simulink model "Experiment_3_cs"  (Simulink 8.4)
settings: Solver=ode5  SolverMode=SingleTasking  StartTime=0.0  StopTime=inf  FixedStep=1/100  RelTol=1e-3
PreLoadFcn:
  | mbxruntime.callbacks.PreLoadFcn(bdroot);
PostLoadFcn:
  | mbxruntime.callbacks.PostLoadFcn(bdroot);
InitFcn:
  | mbxruntime.callbacks.InitFcn(bdroot);
StartFcn:
  | mbxruntime.callbacks.StartFcn(bdroot);
StopFcn:
  | mbxruntime.callbacks.StopFcn(bdroot);
undefined symbols (not defined in the file or in its folder): dfreq, gray, Rec, SDTV, strel
libraries: simulink x88, PreScanSimulinkLibrary x24, simulink_extras x22, visiontextngfix x15, visionconversions x3, PreScanUsefulBlocks x3, visionsinks x2, simulink_need_slupdate x2, visionstatistics x1, visionmorphops x1, visionanalysis x1
(part 5 of 12)

== system Experiment_3_cs/SELF_Audi_A8_1/DISABLED/GND1 ==
  GND_Alt : Constant  Value=0
  GND_Lat : Constant  Value=0
  GND_Long : Constant  Value=0
  GND_OrientationPitch : Constant  Value=0
  GND_OrientationRoll : Constant  Value=0
  GND_OrientationYaw : Constant  Value=0
  GND_PositionX : Constant  Value=0
  GND_PositionY : Constant  Value=0
  GND_PositionZ : Constant  Value=0
  GND_Velocity : Constant  Value=0
  GND_Yaw_rate : Constant  Value=0
  buscreator : BusCreator  Inputs=11  OutDataTypeStr=Bus: PRESCAN_SELFSENSORDATA  NonVirtualBus=on
  bus : Outport  OutDataTypeStr=Bus: PRESCAN_SELFSENSORDATA
  wires:
  GND_PositionX/1 -> buscreator/1  "PositionX"
  GND_PositionY/1 -> buscreator/2  "PositionY"
  GND_PositionZ/1 -> buscreator/3  "PositionZ"
  GND_OrientationRoll/1 -> buscreator/4  "OrientationRoll"
  GND_OrientationPitch/1 -> buscreator/5  "OrientationPitch"
  GND_OrientationYaw/1 -> buscreator/6  "OrientationYaw"
  GND_Velocity/1 -> buscreator/7  "Velocity"
  GND_Yaw_rate/1 -> buscreator/8  "Yaw_rate"
  GND_Lat/1 -> buscreator/9  "Lat"
  GND_Long/1 -> buscreator/10  "Long"
  GND_Alt/1 -> buscreator/11  "Alt"
  buscreator/1 -> bus/1

== system Experiment_3_cs/SELF_BMW_Z3_1/DISABLED/GND1 ==
  GND_Alt : Constant  Value=0
  GND_Lat : Constant  Value=0
  GND_Long : Constant  Value=0
  GND_OrientationPitch : Constant  Value=0
  GND_OrientationRoll : Constant  Value=0
  GND_OrientationYaw : Constant  Value=0
  GND_PositionX : Constant  Value=0
  GND_PositionY : Constant  Value=0
  GND_PositionZ : Constant  Value=0
  GND_Velocity : Constant  Value=0
  GND_Yaw_rate : Constant  Value=0
  buscreator : BusCreator  Inputs=11  OutDataTypeStr=Bus: PRESCAN_SELFSENSORDATA  NonVirtualBus=on
  bus : Outport  OutDataTypeStr=Bus: PRESCAN_SELFSENSORDATA
  wires:
  GND_PositionX/1 -> buscreator/1  "PositionX"
  GND_PositionY/1 -> buscreator/2  "PositionY"
  GND_PositionZ/1 -> buscreator/3  "PositionZ"
  GND_OrientationRoll/1 -> buscreator/4  "OrientationRoll"
  GND_OrientationPitch/1 -> buscreator/5  "OrientationPitch"
  GND_OrientationYaw/1 -> buscreator/6  "OrientationYaw"
  GND_Velocity/1 -> buscreator/7  "Velocity"
  GND_Yaw_rate/1 -> buscreator/8  "Yaw_rate"
  GND_Lat/1 -> buscreator/9  "Lat"
  GND_Long/1 -> buscreator/10  "Long"
  GND_Alt/1 -> buscreator/11  "Alt"
  buscreator/1 -> bus/1

== system Experiment_3_cs/SELF_Male_RegularAni_1/DISABLED/GND1 ==
  GND_Alt : Constant  Value=0
  GND_Lat : Constant  Value=0
  GND_Long : Constant  Value=0
  GND_OrientationPitch : Constant  Value=0
  GND_OrientationRoll : Constant  Value=0
  GND_OrientationYaw : Constant  Value=0
  GND_PositionX : Constant  Value=0
  GND_PositionY : Constant  Value=0
  GND_PositionZ : Constant  Value=0
  GND_Velocity : Constant  Value=0
  GND_Yaw_rate : Constant  Value=0
  buscreator : BusCreator  Inputs=11  OutDataTypeStr=Bus: PRESCAN_SELFSENSORDATA  NonVirtualBus=on
  bus : Outport  OutDataTypeStr=Bus: PRESCAN_SELFSENSORDATA
  wires:
  GND_PositionX/1 -> buscreator/1  "PositionX"
  GND_PositionY/1 -> buscreator/2  "PositionY"
  GND_PositionZ/1 -> buscreator/3  "PositionZ"
  GND_OrientationRoll/1 -> buscreator/4  "OrientationRoll"
  GND_OrientationPitch/1 -> buscreator/5  "OrientationPitch"
  GND_OrientationYaw/1 -> buscreator/6  "OrientationYaw"
  GND_Velocity/1 -> buscreator/7  "Velocity"
  GND_Yaw_rate/1 -> buscreator/8  "Yaw_rate"
  GND_Lat/1 -> buscreator/9  "Lat"
  GND_Long/1 -> buscreator/10  "Long"
  GND_Alt/1 -> buscreator/11  "Alt"
  buscreator/1 -> bus/1

== system Experiment_3_cs/SELF_Nissan_Cabstar_1/DISABLED/GND1 ==
  GND_Alt : Constant  Value=0
  GND_Lat : Constant  Value=0
  GND_Long : Constant  Value=0
  GND_OrientationPitch : Constant  Value=0
  GND_OrientationRoll : Constant  Value=0
  GND_OrientationYaw : Constant  Value=0
  GND_PositionX : Constant  Value=0
  GND_PositionY : Constant  Value=0
  GND_PositionZ : Constant  Value=0
  GND_Velocity : Constant  Value=0
  GND_Yaw_rate : Constant  Value=0
  buscreator : BusCreator  Inputs=11  OutDataTypeStr=Bus: PRESCAN_SELFSENSORDATA  NonVirtualBus=on
  bus : Outport  OutDataTypeStr=Bus: PRESCAN_SELFSENSORDATA
  wires:
  GND_PositionX/1 -> buscreator/1  "PositionX"
  GND_PositionY/1 -> buscreator/2  "PositionY"
  GND_PositionZ/1 -> buscreator/3  "PositionZ"
  GND_OrientationRoll/1 -> buscreator/4  "OrientationRoll"
  GND_OrientationPitch/1 -> buscreator/5  "OrientationPitch"
  GND_OrientationYaw/1 -> buscreator/6  "OrientationYaw"
  GND_Velocity/1 -> buscreator/7  "Velocity"
  GND_Yaw_rate/1 -> buscreator/8  "Yaw_rate"
  GND_Lat/1 -> buscreator/9  "Lat"
  GND_Long/1 -> buscreator/10  "Long"
  GND_Alt/1 -> buscreator/11  "Alt"
  buscreator/1 -> bus/1

== system Experiment_3_cs/TIS_1/DISABLED/GND1 ==
  GND_DATA : Subsystem
  GND_HEADER : Subsystem
  buscreator : BusCreator  Inputs=2  OutDataTypeStr=Bus: PRESCAN_SCANNERSENSOR_MESSAGE  NonVirtualBus=on
  concatenate : Concatenate  NumInputs=5
  bus : Outport  OutDataTypeStr=Bus: PRESCAN_SCANNERSENSOR_MESSAGE
  wires:
  GND_HEADER/1(bus) -> buscreator/1  "HEADER"
  GND_DATA/1(bus) -> buscreator/2  "DATA"
  buscreator/1 -> concatenate/1, concatenate/2, concatenate/3, concatenate/4, concatenate/5
  concatenate/1 -> bus/1

== system Experiment_3_cs/TIS_2/DISABLED/GND1 ==
  GND_DATA : Subsystem
  GND_HEADER : Subsystem
  buscreator : BusCreator  Inputs=2  OutDataTypeStr=Bus: PRESCAN_SCANNERSENSOR_MESSAGE  NonVirtualBus=on
  concatenate : Concatenate  NumInputs=5
  bus : Outport  OutDataTypeStr=Bus: PRESCAN_SCANNERSENSOR_MESSAGE
  wires:
  GND_HEADER/1(bus) -> buscreator/1  "HEADER"
  GND_DATA/1(bus) -> buscreator/2  "DATA"
  buscreator/1 -> concatenate/1, concatenate/2, concatenate/3, concatenate/4, concatenate/5
  concatenate/1 -> bus/1

== system Experiment_3_cs/Actros_2541_1/ENABLED/Dynamics_Empty/MuxState ==
  note: mode: Dynamics
  note: mode: Positioning
  note: mode: Dynamics
      | VelVEHICLE
      | wrt VEH
  note: AnglesVEHICLE
      | wrtGLOB
  note: For state mode 'Dynamic' positions
      | are not taken into account, as they
      | are computed by integrating velocity.
      | Click annotation for Help.
  x [m] : Inport  SampleTime=TimeStep
  y [m] : Inport  Port=2  SampleTime=TimeStep
  z [m] : Inport  Port=3  SampleTime=TimeStep
  dx [m/s] : Inport  Port=4  SampleTime=TimeStep
  dy [m/s] : Inport  Port=5  SampleTime=TimeStep
  dz [m/s] : Inport  Port=6  SampleTime=TimeStep
  R [rad] : Inport  Port=7  SampleTime=TimeStep
  P [rad] : Inport  Port=8  SampleTime=TimeStep
  Y [rad] : Inport  Port=9  SampleTime=TimeStep
  Constant : Constant  DisableCoverage=on  Value=positioningmode
  Discrete-Time Integrator : DiscreteIntegrator  SampleTime=TimeStep
  Ground : Ground
  Ground1 : Ground
  Mux1 : Mux  Inputs=[3 3]
  Mux2 : Mux  Inputs=3
  Mux3 : Mux  Inputs=3
  Mux4 : Mux  Inputs=3
  Mux5 : Mux  Inputs=[3 3]
  Mux6 : Mux  Inputs=[6 3]
  Switch : Switch  Threshold=0.5
  Transformation_BODY2GLOBAL : PreScanSimulinkLibrary/Simple_Vehicle_Dynamics/Chassis/MuxDynState/Transformation_BODY2GLOBAL
  mux3 : Mux  Inputs=3
  state : Outport
  wires:
  Constant/1 -> Switch/2
  Mux6/1 -> state/1
  Mux4/1 -> Mux1/1
  Mux5/1 -> Switch/3
  Mux1/1 -> Switch/1
  Switch/1 -> Mux6/1  "PosVeh wrt  GLOB"
  P [rad]/1 -> Mux3/2
  R [rad]/1 -> Mux3/1
  dz [m/s]/1 -> Mux2/3
  dy [m/s]/1 -> Mux2/2
  dx [m/s]/1 -> Mux2/1
  z [m]/1 -> Mux4/3
  y [m]/1 -> Mux4/2
  x [m]/1 -> Mux4/1
  Ground1/1 -> mux3/2  "pitch"
  Y [rad]/1 -> mux3/3, Mux3/3  "yaw"
  Mux3/1 -> Mux6/2
  Transformation_BODY2GLOBAL/1 -> Discrete-Time Integrator/1, Mux5/2  "VelVEH wrt  GLOB"
  mux3/1 -> Transformation_BODY2GLOBAL/2
  Ground/1 -> mux3/1  "roll"
  Mux2/1 -> Mux1/2, Transformation_BODY2GLOBAL/1
  Discrete-Time Integrator/1 -> Mux5/1  "PosVEH wrt  GLOB"

== system Experiment_3_cs/Actros_2541_1/ENABLED/SELF_Demux/compas converter ==
  rotz [rad] : Inport
  cart2compas : Subsystem
  rad2deg : Gain  Gain=180/pi
  heading [deg] : Outport
  wires:
  rad2deg/1 -> cart2compas/1(Angle [deg])
  rotz [rad]/1 -> rad2deg/1
  cart2compas/1(heading [deg]) -> heading [deg]/1

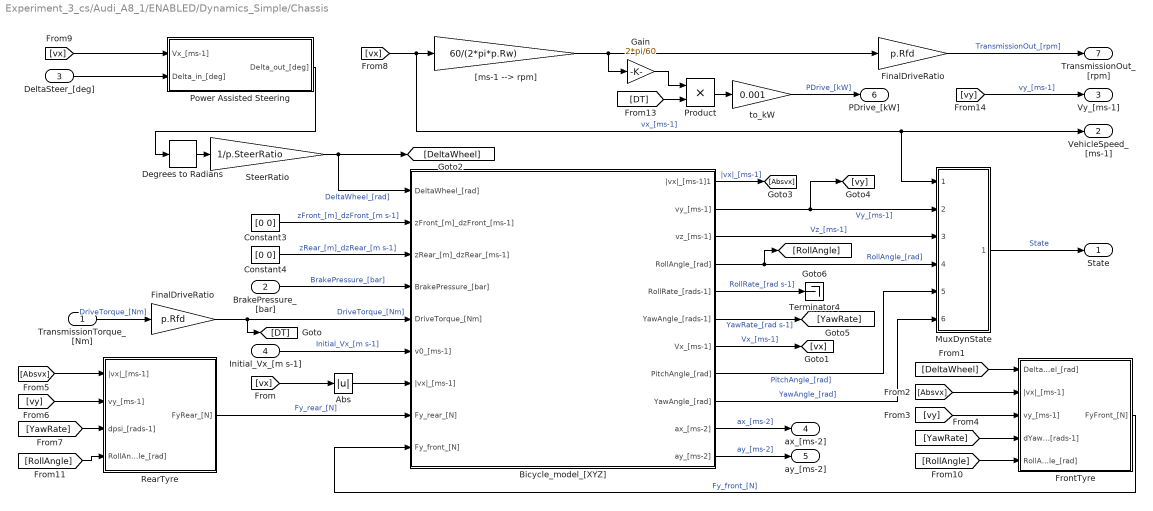
== system Experiment_3_cs/Audi_A8_1/ENABLED/Dynamics_Simple/Chassis ==
  TransmissionTorque_[Nm] : Inport
  BrakePressure_[bar] : Inport  Port=2
  DeltaSteer_[deg] : Inport  Port=3
  Initial_Vx_[m s-1] : Inport  Port=4
  Abs : Abs
  Bicycle_model_[XYZ] : Subsystem
      mask Display: image(imread('Bicycle_model.png'));
  Constant3 : Constant  Value=[0 0]
  Constant4 : Constant  Value=[0 0]
  Degrees to Radians : simulink_extras/Transformations/Degrees to Radians
  FinalDriveRatio : Gain  Gain=p.Rfd  SaturateOnIntegerOverflow=on  OutDataTypeStr=Inherit: Same as input  ParamDataTypeStr=Inherit: Same as input
  "FinalDriveRatio " : Gain  Gain=p.Rfd  SaturateOnIntegerOverflow=on  OutDataTypeStr=Inherit: Same as input  ParamDataTypeStr=Inherit: Same as input
  FrontTyre : Subsystem
      mask Display: image(imread('Tyre.png'));
  Gain : Gain  Gain=2*pi/60
  MuxDynState : Subsystem
  Power Assisted Steering : Subsystem
  Product : Product  RndMeth=Zero
  RearTyre : Subsystem
      mask Display: image(imread('Tyre.png'));
  SteerRatio : Gain  Gain=1/p.SteerRatio
  Terminator4 : Terminator
  "[ms-1 --> rpm]" : Gain  Gain=60/(2*pi*p.Rw)  SaturateOnIntegerOverflow=on  OutDataTypeStr=Inherit: Same as input  ParamDataTypeStr=Inherit: Same as input
  to_kW : Gain  Gain=0.001
  State : Outport
  VehicleSpeed_[ms-1] : Outport  Port=2
  Vy_[ms-1] : Outport  Port=3
  ax_[ms-2] : Outport  Port=4
  ay_[ms-2] : Outport  Port=5
  PDrive_[kW] : Outport  Port=6
  TransmissionOut_[rpm] : Outport  Port=7
  wires:
  [vy] -> Vy_[ms-1]/1  "vy_[ms-1]"
  to_kW/1 -> PDrive_[kW]/1  "PDrive_[kW]"
  Gain/1 -> Product/1
  Bicycle_model_[XYZ]/10(ax_[ms-2]) -> ax_[ms-2]/1  "ax_[ms-2]"
  Product/1 -> to_kW/1
  [DT] -> Product/2
  Bicycle_model_[XYZ]/11(ay_[ms-2]) -> ay_[ms-2]/1  "ay_[ms-2]"
  Abs/1 -> Bicycle_model_[XYZ]/7(|vx|_[ms-1])
  Degrees to Radians/1 -> SteerRatio/1
  [vx] -> Abs/1
  SteerRatio/1 -> [DeltaWheel], Bicycle_model_[XYZ]/1(DeltaWheel_[rad])  "DeltaWheel_[rad]"
  TransmissionTorque_[Nm]/1 -> "FinalDriveRatio "/1  "DriveTorque_[Nm]"
  RearTyre/1(FyRear_[N]) -> Bicycle_model_[XYZ]/8(Fy_rear_[N])  "Fy_rear_[N]"
  FrontTyre/1(FyFront_[N]) -> Bicycle_model_[XYZ]/9(Fy_front_[N])  "Fy_front_[N]"
  Bicycle_model_[XYZ]/1(|vx|_[ms-1]1) -> [Absvx]  "|vx|_[ms-1]"
  Bicycle_model_[XYZ]/2(vy_[ms-1]) -> [vy], MuxDynState/2(vy [ms-1])  "Vy_[ms-1]"
  Bicycle_model_[XYZ]/4(RollAngle_[rad]) -> MuxDynState/4(R [rad]), [RollAngle]  "RollAngle_[rad]"
  Bicycle_model_[XYZ]/6(YawAngle_[rads-1]) -> [YawRate]  "YawRate_[rad s-1]"
  Bicycle_model_[XYZ]/7(Vx_[ms-1]) -> [vx]  "Vx_[ms-1]"
  [DeltaWheel] -> FrontTyre/1(DeltaWheel_[rad])
  [Absvx] -> FrontTyre/2(|vx|_[ms-1])
  [vy] -> FrontTyre/3(vy_[ms-1])
  [YawRate] -> FrontTyre/4(dYawAngle_[rads-1])
  [Absvx] -> RearTyre/1(|vx|_[ms-1])
  [vy] -> RearTyre/2(vy_[ms-1])
  [YawRate] -> RearTyre/3(dpsi_[rads-1])
  Bicycle_model_[XYZ]/3(vz_[ms-1]) -> MuxDynState/3(vz [ms-1])  "Vz_[ms-1]"
  Bicycle_model_[XYZ]/8(PitchAngle_[rad]) -> MuxDynState/5(P [rad])  "PitchAngle_[rad]"
  Bicycle_model_[XYZ]/9(YawAngle_[rad]) -> MuxDynState/6(Y [rad])  "YawAngle_[rad]"
  "[ms-1 --> rpm]"/1 -> Gain/1, FinalDriveRatio/1
  FinalDriveRatio/1 -> TransmissionOut_[rpm]/1  "TransmissionOut_[rpm]"
  [vx] -> "[ms-1 --> rpm]"/1, VehicleSpeed_[ms-1]/1, MuxDynState/1(vx [ms-1])  "vx_[ms-1]"
  [vx] -> Power Assisted Steering/1(Vx_[ms-1])
  DeltaSteer_[deg]/1 -> Power Assisted Steering/2(Delta_in_[deg])
  Power Assisted Steering/1(Delta_out_[deg]) -> Degrees to Radians/1
  [RollAngle] -> FrontTyre/5(RollAngle_[rad])
  [RollAngle] -> RearTyre/4(RollAngle_[rad])
  Constant3/1 -> Bicycle_model_[XYZ]/2(zFront_[m]_dzFront_[ms-1])  "zFront_[m]_dzFront_[m s-1]"
  Constant4/1 -> Bicycle_model_[XYZ]/3(zRear_[m]_dzRear_[ms-1])  "zRear_[m]_dzRear_[m s-1]"
  BrakePressure_[bar]/1 -> Bicycle_model_[XYZ]/4(BrakePressure_[bar])  "BrakePressure_[bar]"
  "FinalDriveRatio "/1 -> Bicycle_model_[XYZ]/5(DriveTorque_[Nm]), [DT]  "DriveTorque_[Nm]"
  Initial_Vx_[m s-1]/1 -> Bicycle_model_[XYZ]/6(v0_[ms-1])  "Initial_Vx_[m s-1]"
  Bicycle_model_[XYZ]/5(RollRate_[rads-1]) -> Terminator4/1  "RollRate_[rad s-1]"
  MuxDynState/1(State) -> State/1  "State"

== system Experiment_3_cs/Audi_A8_1/ENABLED/Dynamics_Simple/Engine ==
  ImpellerTorque_[Nm] : Inport
  Throttle_[%] : Inport  Port=2
  Configurable Subsystem : Subsystem  BlockChoice=Rate Limiter  mask{ComputationMode=ComputationMode}
      mask prompts: ComputationMode "Compuation mode:"
      mask init:
      | SetComputationMode(gcb,ComputationMode);
      settings: AttributesFormatString=%<BlockChoice>  OpenFcn=BringToFront(gcb);  MemberBlocks=Discrete Rate Limiter,Rate Limiter
      settings: TemplateBlock=|
      | PreScanSimulinkLibrary/Configurable Subsystems/TransferFunction
      | Engine/Configurable
      | Subsystem
  Configurable Subsystem1 : Subsystem  BlockChoice=Integrator  mask{ComputationMode=ComputationMode}
      mask prompts: ComputationMode "Computation mode:"
      mask init:
      | SetComputationMode(gcb,ComputationMode);
      settings: AttributesFormatString=%<BlockChoice>  OpenFcn=BringToFront(gcb);  MemberBlocks=Discrete-Time Integrator,Integrator
      settings: TemplateBlock=|
      | PreScanSimulinkLibrary/Configurable Subsystems/integral with initial condition and limts
      | for engine/Configurable
      | Subsystem
  EngineTorque : Lookup2D  RowIndex=p.thvec  ColumnIndex=p.nevec  Table=p.emap  InputSameDT=on
  Gain : Gain  Gain=2*pi/60
  Product : Product  RndMeth=Zero
  Sum : Sum  Inputs=-+  SaturateOnIntegerOverflow=on  InputSameDT=on  OutDataTypeStr=Inherit: Same as first input
  engine + impeller inertia : Gain  Gain=1/p.Iei  SaturateOnIntegerOverflow=on  OutDataTypeStr=Inherit: Same as input  ParamDataTypeStr=Inherit: Same as input
  to_kW : Gain  Gain=0.001
  nEngine_[rpm] : Outport  InitialOutput=0
  PEngine_[kW] : Outport  Port=2  InitialOutput=0
  wires:
  EngineTorque/1 -> Sum/2, Product/2
  engine + impeller inertia/1 -> Configurable Subsystem1/1(In1)
  Sum/1 -> engine + impeller inertia/1
  Configurable Subsystem1/1(Out1) -> nEngine_[rpm]/1, EngineTorque/2, Gain/1  "rpm"
  Throttle_[%]/1 -> Configurable Subsystem/1(In1)
  ImpellerTorque_[Nm]/1 -> Sum/1
  Configurable Subsystem/1(Out1) -> EngineTorque/1
  Product/1 -> to_kW/1
  Gain/1 -> Product/1
  to_kW/1 -> PEngine_[kW]/1

== system Experiment_3_cs/Audi_A8_1/ENABLED/Dynamics_Simple/Gear: Auto Manual ==
  note: 0; Auto = on // Manual =off
      | 1; Auto = off // Manual =on
  Auto_Manual : Inport
  Manual_Gear : Inport  Port=2
  Auto_Gear : Inport  Port=3
  If : If  IfExpression=u1 == 0
  If Action Subsystem : Subsystem  TreatAsAtomicUnit=on
  If Action Subsystem1 : Subsystem  TreatAsAtomicUnit=on
  Merge : Merge
  Gear : Outport
  wires:
  If Action Subsystem/1(Out1) -> Merge/1
  Auto_Gear/1 -> If Action Subsystem/1(In1)
  If/1 -> If Action Subsystem/Action
  Merge/1 -> Gear/1
  If Action Subsystem1/1(Out1) -> Merge/2
  Manual_Gear/1 -> If Action Subsystem1/1(In1)
  If/2 -> If Action Subsystem1/Action
  Auto_Manual/1 -> If/1

== system Experiment_3_cs/Audi_A8_1/ENABLED/Dynamics_Simple/ShiftLogic ==
  Throttle_[%] : Inport
  GearNr_[-] : Inport  Port=2
  Auto_GearShift : Inport  Port=3
  VehSpeed_[ms-1] : Inport  Port=4
  Add2 : Sum
  Data Type Conversion1 : DataTypeConversion  OutDataTypeStr=double
  Detect Increase1 : simulink/Logic and Bit Operations/Detect Increase  vinit=0.0  InputProcessing=Inherited  OutDataTypeStr=uint8
  Detect Increase : Subsystem
  Gear limitation : Saturate  UpperLimit=p.maxGear  LowerLimit=1
  Gear limitation while shifting : Saturate  UpperLimit=p.maxGear  LowerLimit=1
  GearNeutral : Constant  Value=0
  GearReverse : Constant  Value=-1
  "IC, gear = 1" : Memory  X0=1  InheritSampleTime=on
  If Action Neutral : Subsystem  TreatAsAtomicUnit=on
  If Action Normal : Subsystem  TreatAsAtomicUnit=on
  If Action Reverse : Subsystem  TreatAsAtomicUnit=on
  Memory : Memory  InheritSampleTime=on
  Merge : Merge  Inputs=3
  Relational Operator : RelationalOperator  OutDataTypeStr=boolean
  Relational Operator1 : RelationalOperator  Operator=<=  OutDataTypeStr=boolean
  Shift_Down time : Delay  DelayLength=p.ShiftDown_fac  InputProcessing=Inherited
  Shift_Up time : Delay  DelayLength=p.ShiftUp_fac  InputProcessing=Inherited
  Sum : Sum  Inputs=+-
  interp_down : Lookup2D  RowIndex=p.downth  ColumnIndex=[1:p.maxGear]  Table=p.downtab  LookUpMeth=Interpolation-Use End Values  InputSameDT=on
  interp_up : Lookup2D  RowIndex=p.upth  ColumnIndex=[1:p.maxGear]  Table=p.uptab  LookUpMeth=Interpolation-Use End Values  InputSameDT=on
  reverse/neutral/normal gear : If  IfExpression=u1 == 0  ElseIfExpressions=u1 < 0
  to_ms-1 : Gain  Gain=1/3.6
  "to_ms-1 " : Gain  Gain=1/3.6
  GearNr : Outport
  wires:
  Auto_GearShift/1 -> reverse/neutral/normal gear/1
  "IC, gear = 1"/1 -> If Action Normal/1(In1)
  Merge/1 -> GearNr/1
  If Action Reverse/1(Out1) -> Merge/2
  If Action Neutral/1(Out1) -> Merge/1
  If Action Normal/1(Out1) -> Merge/3
  reverse/neutral/normal gear/3 -> If Action Normal/Action
  reverse/neutral/normal gear/1 -> If Action Neutral/Action
  reverse/neutral/normal gear/2 -> If Action Reverse/Action
  GearReverse/1 -> If Action Reverse/1(In1)
  GearNeutral/1 -> If Action Neutral/1(In1)
  Shift_Down time/1 -> Sum/2
  Shift_Up time/1 -> Sum/1
  Detect Increase/1(Out1) -> Shift_Up time/1
  Data Type Conversion1/1 -> Shift_Down time/1
  Detect Increase1/1 -> Data Type Conversion1/1
  Sum/1 -> Add2/1
  Memory/1 -> Add2/2  "GearNr_[-]"
  Add2/1 -> Gear limitation while shifting/1
  Gear limitation while shifting/1 -> "IC, gear = 1"/1, Memory/1  "GearNr_[-]"
  Throttle_[%]/1 -> interp_down/1, interp_up/1
  Relational Operator/1 -> Detect Increase/2(In2)
  Relational Operator1/1 -> Detect Increase1/1
  interp_down/1 -> "to_ms-1 "/1
  VehSpeed_[ms-1]/1 -> Relational Operator/1, Relational Operator1/1
  interp_up/1 -> to_ms-1/1
  Gear limitation/1 -> interp_down/2, interp_up/2, Detect Increase/1(GearNr_[-])
  GearNr_[-]/1 -> Gear limitation/1
  to_ms-1/1 -> Relational Operator/2
  "to_ms-1 "/1 -> Relational Operator1/2

== system Experiment_3_cs/Audi_A8_1/ENABLED/Dynamics_Simple/Transmission ==
  nEngine_[rpm] : Inport
  GearNr_[-] : Inport  Port=2
  n_TransmissionOut_[rpm] : Inport  Port=3
  Torque_Converter : Subsystem
      mask Display: image(imread('TorqueConverter.png'));
  Transmission_Ratio : Subsystem
  Viscous coupling : Lookup  InputValues=[-5:0.1:5]*p.m/4  Table=p.m/4*tanh([-5:0.1:5])
  ImpellerTorque_[Nm] : Outport  InitialOutput=0
  TransmissionTorque_[Nm] : Outport  Port=2  InitialOutput=0
  wires:
  Torque_Converter/2(TurbineTorque_[Nm]) -> Viscous coupling/1  "Converter_Torque_[Nm]"
  Transmission_Ratio/2(nTransmissionIn_[rpm]) -> Torque_Converter/2(nTransmission_[rpm])
  nEngine_[rpm]/1 -> Torque_Converter/1(nEngine_[rpm])
  GearNr_[-]/1 -> Transmission_Ratio/2(GearNr_[-]), Torque_Converter/3(Gear nr)
  n_TransmissionOut_[rpm]/1 -> Transmission_Ratio/3(nTransmissionOut_[rpm])
  Torque_Converter/1(ImpellerTorque_[Nm]) -> ImpellerTorque_[Nm]/1
  Transmission_Ratio/1(tTransmissionOut_[Nm]) -> TransmissionTorque_[Nm]/1
  Viscous coupling/1 -> Transmission_Ratio/1(tTransmissionIn_[Nm])

== system Experiment_3_cs/Audi_A8_1/ENABLED/PPS Model/Actuation ==
  Flag0.6 : Inport
  Det flag : Inport  Port=2
  Flag1.6 : Inport  Port=3
  brake dem : Inport  Port=4
  throttle dem : Inport  Port=5
  Pedestrian detection : Inport  Port=6
  Braking Lights : Subsystem
  Compare To Zero : simulink/Logic and Bit Operations/Compare To Zero  relop=>  OutDataTypeStr=uint8
  Constant : Constant  Value=MaxBrakePressure  SampleTime=[0,0]
  Constant1 : Constant  Value=0  SampleTime=[0,0]
  Data Store Read : DataStoreRead  DataStoreName=full_brake  SampleTime=1/Mainfreq
  Display1 : Display
  If : If  IfExpression=u1  ShowElse=off
  If Action Subsystem : Subsystem  TreatAsAtomicUnit=on
  Logical Operator : Logic  AllPortsSameDT=off  OutDataTypeStr=boolean  SampleTime=[0,0]
  Logical Operator1 : Logic  Operator=OR  AllPortsSameDT=off  OutDataTypeStr=boolean  SampleTime=[0,0]
  Logical Operator2 : Logic  AllPortsSameDT=off  OutDataTypeStr=boolean  SampleTime=[0,0]
  Logical Operator3 : Logic  AllPortsSameDT=off  OutDataTypeStr=boolean  SampleTime=1/TISfreq
  Logical Operator4 : Logic  AllPortsSameDT=off  OutDataTypeStr=boolean  SampleTime=1/TISfreq
  Logical Operator5 : Logic  Operator=OR  AllPortsSameDT=off  OutDataTypeStr=boolean  SampleTime=1/TISfreq
  Logical Operator6 : Logic  Operator=OR  AllPortsSameDT=off  OutDataTypeStr=boolean  SampleTime=1/TISfreq
  Rate Limiter : RateLimiter  RisingSlewLimit=1000*0.9*MaxBrakePressure/BrakeDelay  FallingSlewLimit=-inf  SampleTimeMode=inherited
  Rate Transition1 : RateTransition  Integrity=off  OutPortSampleTime=[0,0]
  Rate Transition2 : RateTransition  Integrity=off  OutPortSampleTime=[0,0]
  Rate Transition3 : RateTransition  Integrity=off  OutPortSampleTime=[0,0]
  Switch1 : Switch  Criteria=u2 > Threshold  SampleTime=[0,0]
  Switch3 : Switch  Criteria=u2 > Threshold  SampleTime=[0,0]
  Switch4 : Switch  Criteria=u2 > Threshold  SampleTime=[0,0]
  Terminator_1 : Terminator
  brake : Outport  SampleTime=[0,0]
  throttle : Outport  Port=2  SampleTime=[0,0]
  BrakeLights : Outport  Port=3  SampleTime=1/Mainfreq
  Warning flag : Outport  Port=4
  Detection flag : Outport  Port=5
  Braking flag : Outport  Port=6
  wires:
  Logical Operator1/1 -> Logical Operator/2
  Logical Operator2/1 -> Logical Operator1/2
  Compare To Zero/1 -> Logical Operator2/2
  Constant/1 -> Switch3/1
  Constant1/1 -> Switch4/1
  Switch4/1 -> throttle/1
  throttle dem/1 -> Switch4/3
  Braking Lights/1(BrakeLights (3x1)) -> BrakeLights/1
  brake dem/1 -> Rate Transition1/1
  Rate Transition1/1 -> Compare To Zero/1, Switch3/3
  Rate Transition2/1 -> Logical Operator2/1
  Rate Transition3/1 -> Logical Operator1/1
  Switch3/1 -> Switch1/3, Rate Limiter/1
  Rate Limiter/1 -> Switch1/1
  Switch1/1 -> brake/1
  Logical Operator3/1 -> Rate Transition3/1, Braking flag/1, Logical Operator6/1, Logical Operator5/1
  Logical Operator4/1 -> Rate Transition2/1, Logical Operator6/2
  Flag0.6/1 -> Logical Operator3/2
  Flag1.6/1 -> Logical Operator4/2
  Logical Operator6/1 -> Warning flag/1
  Logical Operator5/1 -> Detection flag/1
  Logical Operator/1 -> If/1
  Data Store Read/1 -> Braking Lights/1(switcher), Switch4/2, Switch3/2, Switch1/2
  If/1 -> If Action Subsystem/Action
  Det flag/1 -> Logical Operator4/1, Logical Operator/1, Logical Operator3/1, Display1/1, Logical Operator5/2
  Pedestrian detection/1 -> Terminator_1/1

== system Experiment_3_cs/Audi_A8_1/ENABLED/PPS Model/PPS EGO State Display ==
  V [km/h] : Inport
  RPM : Inport  Port=2
  Ax : Inport  Port=3  SampleTime=[0,0]
  Brake Pressure [bar] : Inport  Port=4
  Warning flag : Inport  Port=5  OutDataTypeStr=boolean
  Detection flag : Inport  Port=6  OutDataTypeStr=boolean
  Braking flag : Inport  Port=7  OutDataTypeStr=boolean
  Ped det flag : Inport  Port=8  OutDataTypeStr=boolean
  TTC : Inport  Port=9
  cd : Inport  Port=10  OutDataTypeStr=boolean
  Constant : Constant  Value=DisplaySwitch
  Data Type Conversion{,1..3} (4 alike) : DataTypeConversion  OutDataTypeStr=boolean
  Detect Rise Positive1 : simulink/Logic and Bit Operations/Detect Rise Positive  vinit=0  InputProcessing=Inherited  OutDataTypeStr=uint8
  Detect Rise Positive4 : simulink/Logic and Bit Operations/Detect Rise Positive  vinit=0  InputProcessing=Inherited  OutDataTypeStr=uint8
  Display function : Subsystem
  Plots : Subsystem
      mask help:
      | The block calls functions:
      | * PPS_Speed_Profile
      | * PPS_TTC_Profile
      | to generate plots at the end of the simulation.
      | See stop callback of the block for more details.
  Rate Transition{,1..2,5,7..8} (6 alike) : RateTransition  Integrity=off  OutPortSampleTime=1/DisplayFreq
  Rate Transition10 : RateTransition  Integrity=off  OutPortSampleTime=[0,0]
  Rate Transition3 : RateTransition  Integrity=off  OutPortSampleTime=[0,0]
  Rate Transition4 : RateTransition  Integrity=off  OutPortSampleTime=1/Mainfreq
  Rate Transition6 : RateTransition  Integrity=off  OutPortSampleTimeOpt=Inherit  OutPortSampleTime=1/dfreq
  Rate Transition9 : RateTransition  Integrity=off  OutPortSampleTime=1/Mainfreq
  Switch : Switch  Criteria=u2 > Threshold  SampleTime=1/Mainfreq
  Switch1 : Switch  Criteria=u2 > Threshold  SampleTime=1/Mainfreq
  To Workspace1 : ToWorkspace  VariableName=VRU_EGO_State_Coll  SampleTime=1/Mainfreq
      settings: MaxDataPoints=1
  To Workspace2 : ToWorkspace  VariableName=VRU_DisplaySwitch  SampleTime=1/Mainfreq
      settings: MaxDataPoints=1
  Unit Delay : UnitDelay  SampleTime=1/Mainfreq
  Unit Delay1 : UnitDelay  SampleTime=-1
  Unit Delay2 : UnitDelay  SampleTime=1/Mainfreq
  wires:
  RPM/1 -> Rate Transition1/1
  Brake Pressure [bar]/1 -> Rate Transition2/1
  V [km/h]/1 -> Rate Transition/1, Rate Transition4/1
  Warning flag/1 -> Data Type Conversion1/1
  Ped det flag/1 -> Data Type Conversion3/1
  TTC/1 -> Rate Transition8/1
  Detection flag/1 -> Data Type Conversion/1
  Rate Transition/1 -> Display function/1(V [km/h]), Plots/1(V), Switch1/1
  Rate Transition1/1 -> Display function/2(RPM)
  Rate Transition3/1 -> To Workspace1/1
  cd/1 -> Rate Transition9/1
  Switch/1 -> Unit Delay/1, Rate Transition3/1
  Unit Delay/1 -> Switch/3
  Rate Transition4/1 -> Switch/1
  Detect Rise Positive4/1 -> Switch/2
  Braking flag/1 -> Rate Transition5/1
  Rate Transition5/1 -> Data Type Conversion2/1, Detect Rise Positive1/1
  Ax/1 -> Rate Transition6/1
  Unit Delay1/1 -> Rate Transition7/1
  Rate Transition6/1 -> Unit Delay1/1
  Rate Transition2/1 -> Display function/3(Brake Pressure)
  Rate Transition7/1 -> Plots/2(Ax)
  Rate Transition8/1 -> Plots/7(ttc), Display function/8(TTC)
  Rate Transition9/1 -> Detect Rise Positive4/1
  Data Type Conversion3/1 -> Plots/6(ped), Display function/7(Pet det flag)
  Data Type Conversion2/1 -> Display function/6(Braking flag), Plots/5(brake)
  Data Type Conversion1/1 -> Plots/4(warn), Display function/5(Warning Flag)
  Data Type Conversion/1 -> Plots/3(det), Display function/4(Detection flag)
  Constant/1 -> Display function/Enable, To Workspace2/1
  Detect Rise Positive1/1 -> Switch1/2
  Switch1/1 -> Unit Delay2/1, Rate Transition10/1
  Unit Delay2/1 -> Switch1/3
  Rate Transition10/1 -> Plots/8(Coll)

== system Experiment_3_cs/Audi_A8_1/ENABLED/PPS Model/PPS_Radar ==
  Range : Inport
  Theta : Inport  Port=2
  All flags : Inport  Port=3  OutDataTypeStr=boolean
  Flag 0.6 : Inport  Port=4  OutDataTypeStr=boolean
  Constant : Constant  Value=RadarSwitch
  Radar : Subsystem
  Rate Transition{1..4} (4 alike) : RateTransition  Integrity=off  Deterministic=off  OutPortSampleTime=1/RadarFreq
  wires:
  Range/1 -> Rate Transition1/1
  Theta/1 -> Rate Transition2/1
  All flags/1 -> Rate Transition3/1
  Flag 0.6/1 -> Rate Transition4/1
  Rate Transition1/1 -> Radar/1(Range)
  Rate Transition2/1 -> Radar/2(Theta)
  Rate Transition3/1 -> Radar/3(All flags)
  Rate Transition4/1 -> Radar/4(Flag 0.6)
  Constant/1 -> Radar/Enable

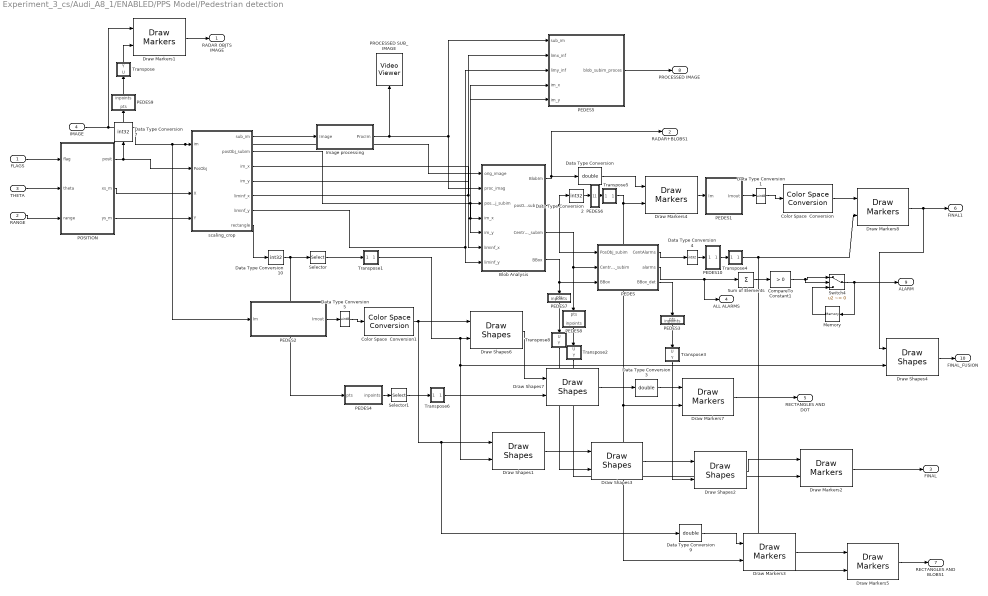
== system Experiment_3_cs/Audi_A8_1/ENABLED/PPS Model/Pedestrian detection ==
  FLAGS : Inport  OutDataTypeStr=boolean
  RANGE : Inport  Port=2  PortDimensions=TISdet
  THETA : Inport  Port=3
  IMAGE : Inport  Port=4  OutDataTypeStr=uint8  PortDimensions=[375 500]
  Blob Analysis : Subsystem
  Color Space  Conversion : visionconversions/Color Space  Conversion  conversion=Obsolete  conversionActive=Y'CbCr to R'G'B'  wp_str=D65  rec=Rec. 601 (SDTV)  sys=1125/60/2:1  imagePorts=One multidimensional signal
  Color Space  Conversion1 : visionconversions/Color Space  Conversion  conversion=Obsolete  conversionActive=Y'CbCr to R'G'B'  wp_str=D65  rec=Rec. 601 (SDTV)  sys=1125/60/2:1  imagePorts=One multidimensional signal
  CompareTo Constant1 : simulink/Logic and Bit Operations/Compare To Constant  relop=>  const=0  OutDataTypeStr=uint8
  Data Type Conversion : DataTypeConversion  OutDataTypeStr=double
  Data Type Conversion1 : DataTypeConversion  OutDataTypeStr=uint8
  Data Type Conversion{2,4,7,10} (4 alike) : DataTypeConversion  OutDataTypeStr=int32
  Data Type Conversion3 : DataTypeConversion  OutDataTypeStr=double
  Data Type Conversion5 : DataTypeConversion  OutDataTypeStr=uint8
  Data Type Conversion9 : DataTypeConversion  OutDataTypeStr=double
  Draw Markers1 : visiontextngfix/Draw Markers  shape=Circle  size=6  fill=on  fillClrSource=Specify via dialog  display=White  intensity=200  color=[200 255 100]  opacity=1  viewport=Entire image  antialiasing=on  inType=Obsolete  imagePorts=One multidimensional signal  prodOutputMode=Binary point scaling  prodOutputWordLength=32  prodOutputFracLength=14  memoryMode=Specify word length  memoryWordLength=16  memoryFracLength=14  roundingMode=Floor  overflowMode=off
  Draw Markers2 : visiontextngfix/Draw Markers  shape=X-mark  size=3  fill=on  fillClrSource=Specify via dialog  display=White  intensity=200  color=[200 255 100]  opacity=0.9  viewport=Entire image  antialiasing=on  inType=Obsolete  imagePorts=One multidimensional signal  prodOutputMode=Binary point scaling  prodOutputWordLength=32  prodOutputFracLength=14  memoryMode=Specify word length  memoryWordLength=16  memoryFracLength=14  roundingMode=Floor  overflowMode=off
  Draw Markers3 : visiontextngfix/Draw Markers  shape=Circle  size=6  fill=on  fillClrSource=Specify via dialog  display=White  intensity=200  color=[255 0 0]  opacity=0.9  viewport=Entire image  antialiasing=on  inType=Obsolete  imagePorts=One multidimensional signal  prodOutputMode=Binary point scaling  prodOutputWordLength=32  prodOutputFracLength=14  memoryMode=Specify word length  memoryWordLength=16  memoryFracLength=14  roundingMode=Floor  overflowMode=off
  Draw Markers4 : visiontextngfix/Draw Markers  shape=Circle  size=6  fill=on  fillClrSource=Specify via dialog  display=White  intensity=200  color=[200 255 100]  opacity=0.9  viewport=Entire image  antialiasing=on  inType=Obsolete  imagePorts=One multidimensional signal  prodOutputMode=Binary point scaling  prodOutputWordLength=32  prodOutputFracLength=14  memoryMode=Specify word length  memoryWordLength=16  memoryFracLength=14  roundingMode=Floor  overflowMode=off
  Draw Markers5 : visiontextngfix/Draw Markers  shape=Circle  size=6  fill=on  fillClrSource=Specify via dialog  display=User-specified value  intensity=200  color=[255 0 0]  opacity=1  viewport=Entire image  antialiasing=on  inType=Obsolete  imagePorts=One multidimensional signal  prodOutputMode=Binary point scaling  prodOutputWordLength=32  prodOutputFracLength=14  memoryMode=Specify word length  memoryWordLength=16  memoryFracLength=14  roundingMode=Floor  overflowMode=off
  Draw Markers7 : visiontextngfix/Draw Markers  shape=Circle  size=6  fill=on  fillClrSource=Specify via dialog  display=White  intensity=200  color=[200 255 100]  opacity=0.9  viewport=Entire image  antialiasing=on  inType=Obsolete  imagePorts=One multidimensional signal  prodOutputMode=Binary point scaling  prodOutputWordLength=32  prodOutputFracLength=14  memoryMode=Specify word length  memoryWordLength=16  memoryFracLength=14  roundingMode=Floor  overflowMode=off
  Draw Markers8 : visiontextngfix/Draw Markers  shape=Circle  size=6  fill=on  fillClrSource=Specify via dialog  display=User-specified value  intensity=200  color=[255 0 0]  opacity=1  viewport=Entire image  antialiasing=on  inType=Obsolete  imagePorts=One multidimensional signal  prodOutputMode=Binary point scaling  prodOutputWordLength=32  prodOutputFracLength=14  memoryMode=Specify word length  memoryWordLength=16  memoryFracLength=14  roundingMode=Floor  overflowMode=off
  Draw Shapes1 : visiontextngfix/Draw Shapes  shape=Rectangles  fill=off  lineWidth=1  fillClrSource=Specify via dialog  display=White  intensity=200  color=[255 0 0]  opacity=0.5  viewport=Entire image  antialiasing=off  inType=Obsolete  imagePorts=One multidimensional signal  prodOutputMode=Binary point scaling  prodOutputWordLength=32  prodOutputFracLength=14  memoryMode=Specify word length  memoryWordLength=16  memoryFracLength=14  roundingMode=Floor  overflowMode=off
  Draw Shapes2 : visiontextngfix/Draw Shapes  shape=Rectangles  fill=on  lineWidth=1  fillClrSource=Specify via dialog  display=White  intensity=200  color=[255 0 0]  opacity=0.5  viewport=Entire image  antialiasing=off  inType=Obsolete  imagePorts=One multidimensional signal  prodOutputMode=Binary point scaling  prodOutputWordLength=32  prodOutputFracLength=14  memoryMode=Specify word length  memoryWordLength=16  memoryFracLength=14  roundingMode=Floor  overflowMode=off
  Draw Shapes3 : visiontextngfix/Draw Shapes  shape=Rectangles  fill=off  lineWidth=1  fillClrSource=Specify via dialog  display=User-specified value  intensity=200  color=[255 0 0]  opacity=0.5  viewport=Entire image  antialiasing=off  inType=Obsolete  imagePorts=One multidimensional signal  prodOutputMode=Binary point scaling  prodOutputWordLength=32  prodOutputFracLength=14  memoryMode=Specify word length  memoryWordLength=16  memoryFracLength=14  roundingMode=Floor  overflowMode=off
  Draw Shapes4 : visiontextngfix/Draw Shapes  shape=Rectangles  fill=off  lineWidth=1  fillClrSource=Specify via dialog  display=White  intensity=200  color=[255 0 0]  opacity=0.5  viewport=Entire image  antialiasing=off  inType=Obsolete  imagePorts=One multidimensional signal  prodOutputMode=Binary point scaling  prodOutputWordLength=32  prodOutputFracLength=14  memoryMode=Specify word length  memoryWordLength=16  memoryFracLength=14  roundingMode=Floor  overflowMode=off
  Draw Shapes6 : visiontextngfix/Draw Shapes  shape=Rectangles  fill=off  lineWidth=1  fillClrSource=Specify via dialog  display=User-specified value  intensity=200  color=[255 0 0]  opacity=0.6  viewport=Entire image  antialiasing=off  inType=Obsolete  imagePorts=One multidimensional signal  prodOutputMode=Binary point scaling  prodOutputWordLength=32  prodOutputFracLength=14  memoryMode=Specify word length  memoryWordLength=16  memoryFracLength=15  roundingMode=Floor  overflowMode=off
  Draw Shapes7 : visiontextngfix/Draw Shapes  shape=Rectangles  fill=on  lineWidth=1  fillClrSource=Specify via dialog  display=White  intensity=200  color=[255 0 0]  opacity=0.5  viewport=Entire image  antialiasing=off  inType=Obsolete  imagePorts=One multidimensional signal  prodOutputMode=Binary point scaling  prodOutputWordLength=32  prodOutputFracLength=14  memoryMode=Specify word length  memoryWordLength=16  memoryFracLength=14  roundingMode=Floor  overflowMode=off
  Image processing : Subsystem
  Memory : Memory
  PEDES : MATLAB Function  TreatAsAtomicUnit=on
  PEDES1 : MATLAB Function  TreatAsAtomicUnit=on
  PEDES10 : MATLAB Function  TreatAsAtomicUnit=on
  PEDES2 : MATLAB Function  TreatAsAtomicUnit=on
  PEDES3 : MATLAB Function  TreatAsAtomicUnit=on
  PEDES4 : MATLAB Function  TreatAsAtomicUnit=on
  PEDES5 : MATLAB Function  TreatAsAtomicUnit=on
  PEDES6 : MATLAB Function  TreatAsAtomicUnit=on
  PEDES7 : MATLAB Function  TreatAsAtomicUnit=on
  PEDES8 : MATLAB Function  TreatAsAtomicUnit=on
  PEDES9 : MATLAB Function  TreatAsAtomicUnit=on
  POSITION : MATLAB Function  TreatAsAtomicUnit=on
  PROCESSED SUB_IMAGE : visionsinks/Video Viewer  inputType=Obsolete7b  imagePorts=One multidimensional signal  useColorMap=off  colormapValue=gray(256)  specRange=off  minInputVal=0  maxInputVal=255  FigPos=[1290 953 500 324]  AxisZoom=on  trueSizedOnce=off  OpenAtMdlStart=on  DefaultConfigurationName=vipscopes.VideoViewerScopeCfg
  Selector : Selector  InputPortWidth=4  Indices=[2, 1, 4, 3]
  Selector1 : Selector  InputPortWidth=4  Indices=[2, 1, 4, 3]
  Sum of Elements : Sum  Inputs=+
  Switch4 : Switch  Criteria=u2 ~= 0
  Transpose : Subsystem
  Transpose1 : Subsystem
  Transpose2 : Subsystem
  Transpose3 : Subsystem
  Transpose4 : Subsystem
  Transpose5 : Subsystem
  Transpose6 : Subsystem
  Transpose8 : Subsystem
  scaling_crop : MATLAB Function  TreatAsAtomicUnit=on
  RADAR OBJTS IMAGE : Outport
  RADAR+BLOBS1 : Outport  Port=2
  FINAL : Outport  Port=3
  ALL ALARMS : Outport  Port=4
  RECTANGLES AND DOT : Outport  Port=5
  FINAL1 : Outport  Port=6
  RECTANGLES AND BLOBS1 : Outport  Port=7
  PROCESSED IMAGE : Outport  Port=8
  ALARM : Outport  Port=9
  FINAL_FUSION : Outport  Port=10
  wires:
  THETA/1 -> POSITION/2(theta)
  FLAGS/1 -> POSITION/1(flag)
  RANGE/1 -> POSITION/3(range)
  Blob Analysis/1(BlobIm) -> RADAR+BLOBS1/1, Data Type Conversion/1
  Blob Analysis/3(Centroid_subim) -> PEDES/2(Centroid_subim), PEDES8/1(pts)
  PEDES/2(alarms) -> ALL ALARMS/1, Sum of Elements/1
  PEDES/1(CentAlarms) -> Data Type Conversion4/1
  Blob Analysis/4(BBox) -> PEDES/3(BBox), PEDES7/1(pts)
  Draw Markers4/1 -> PEDES1/1(Im)
  Data Type Conversion4/1 -> PEDES10/1(pts)
  Color Space  Conversion/1 -> Draw Markers8/1
  PEDES1/1(Imout) -> Data Type Conversion1/1
  Data Type Conversion1/1 -> Color Space  Conversion/1
  Data Type Conversion2/1 -> PEDES6/1(pts)
  Switch4/1 -> Memory/1, ALARM/1
  Memory/1 -> Switch4/3
  Sum of Elements/1 -> CompareTo Constant1/1
  CompareTo Constant1/1 -> Switch4/1, Switch4/2
  Blob Analysis/2(posObj_subim1) -> Data Type Conversion2/1, PEDES/1(PosObj_subim)
  scaling_crop/6(liminf_y) -> PEDES5/3(limy_inf), Blob Analysis/7(liminf_y)
  scaling_crop/7(rectangle) -> Data Type Conversion10/1
  PEDES2/1(Imout) -> Data Type Conversion5/1
  Data Type Conversion5/1 -> Color Space  Conversion1/1
  Color Space  Conversion1/1 -> Draw Shapes6/1, Data Type Conversion9/1, Draw Shapes1/1
  Draw Shapes6/1 -> Draw Shapes7/1
  Draw Shapes7/1 -> Data Type Conversion3/1
  Draw Markers7/1 -> RECTANGLES AND DOT/1
  Draw Shapes1/1 -> Draw Shapes3/1
  Draw Shapes3/1 -> Draw Shapes2/1
  Draw Shapes2/1 -> Draw Markers2/1
  Draw Markers3/1 -> Draw Markers5/1
  Draw Markers5/1 -> RECTANGLES AND BLOBS1/1
  PEDES5/1(blob_subim_proces) -> PROCESSED IMAGE/1
  Draw Markers8/1 -> FINAL1/1, Draw Shapes4/1
  Draw Shapes4/1 -> FINAL_FUSION/1
  Data Type Conversion7/1 -> PEDES9/1(pts)
  POSITION/2(xs_m) -> scaling_crop/3(X)
  Draw Markers1/1 -> RADAR OBJTS IMAGE/1
  POSITION/3(ys_m) -> scaling_crop/4(Y)
  POSITION/1(posit) -> scaling_crop/2(PosObj), Data Type Conversion7/1
  IMAGE/1 -> Blob Analysis/1(orig_image), scaling_crop/1(im), PEDES2/1(Im), Draw Markers1/1
  scaling_crop/1(sub_im) -> Image processing/1(Image)
  scaling_crop/2(posObj_subim) -> Blob Analysis/3(posObj_subim)
  scaling_crop/3(im_x) -> PEDES5/4(im_x), Blob Analysis/4(im_x)
  scaling_crop/4(im_y) -> PEDES5/5(im_y), Blob Analysis/5(im_y)
  scaling_crop/5(liminf_x) -> Blob Analysis/6(liminf_x), PEDES5/2(limx_inf)
  PEDES/3(BBox_det) -> PEDES3/1(pts)
  Draw Markers2/1 -> FINAL/1
  Image processing/1(ProcIm) -> PEDES5/1(sub_im), Blob Analysis/2(proc_imag), PROCESSED SUB_IMAGE/1
  Data Type Conversion/1 -> Draw Markers4/1
  Data Type Conversion9/1 -> Draw Markers3/1
  Data Type Conversion3/1 -> Draw Markers7/1
  Transpose/1(Y) -> Draw Markers1/2
  Transpose1/1(Y) -> Draw Shapes4/2, Draw Shapes1/2, Draw Shapes6/2
  Selector/1 -> Transpose1/1(U)
  Transpose4/1(Y) -> Draw Markers8/2, Draw Markers5/2
  Data Type Conversion10/1 -> Selector/1, PEDES4/1(pts)
  PEDES4/1(inpoints) -> Selector1/1
  Selector1/1 -> Transpose6/1(U)
  Transpose6/1(Y) -> Draw Shapes7/2
  PEDES6/1(inpoints) -> Transpose5/1(U)
  Transpose5/1(Y) -> Draw Markers7/2, Draw Markers3/2, Draw Markers4/2
  PEDES9/1(inpoints) -> Transpose/1(U)
  PEDES10/1(inpoints) -> Transpose4/1(U)
  Transpose3/1(Y) -> Draw Shapes2/2
  Transpose2/1(Y) -> Draw Markers2/2
  Transpose8/1(Y) -> Draw Shapes3/2
  PEDES7/1(inpoints) -> Transpose8/1(U)
  PEDES8/1(inpoints) -> Transpose2/1(U)
  PEDES3/1(inpoints) -> Transpose3/1(U)

== system Experiment_3_cs/Audi_A8_1/ENABLED/PPS Model/Radar detection ==
  EGO_velocity [m/s] : Inport
  EGO_yaw_rate_[deg/s] : Inport  Port=2
  TIS_range [m] : Inport  Port=3  PortDimensions=TISdet
  TIS_rangedot [m/s] : Inport  Port=4  PortDimensions=TISdet
  TIS_theta [deg] : Inport  Port=5  PortDimensions=TISdet
  ind flag : Inport  Port=6
  Abs : Abs
  Bend road segment : Subsystem  TreatAsAtomicUnit=on
  Compare To Constant : simulink/Logic and Bit Operations/Compare To Constant  relop=<=  const=MaxSpeed/3.6  OutDataTypeStr=uint8
  Constant : Constant  Value=2.0
  Constant2 : Constant  Value=1.0
  Data Store Read : DataStoreRead  DataStoreName=full_brake  SampleTime=1/Mainfreq
  Data Type Conversion : DataTypeConversion  OutDataTypeStr=double
  EGO_velocity [m/s]1 : InportShadow
  EGO_yaw_rate_[deg/s]_1 : InportShadow  Port=2
  If : If  IfExpression=u1 > 1  SampleTime=1/TISfreq
  Logical Operator1 : Logic  Operator=NOT  AllPortsSameDT=off  OutDataTypeStr=boolean
  Merge{1..4} (4 alike) : Merge
  Radians to Degrees : simulink_extras/Transformations/Radians to Degrees
  Straight road segment : Subsystem  TreatAsAtomicUnit=on
  Switch : Switch  Criteria=u2 > Threshold
  TIS1 Sorting  Fun : Subsystem
  change lane : Logic  Inputs=3  AllPortsSameDT=off  OutDataTypeStr=boolean
  change lane1 : Logic  Inputs=3  AllPortsSameDT=off  OutDataTypeStr=boolean
  change lane2 : Logic  Inputs=3  AllPortsSameDT=off  OutDataTypeStr=boolean
  TTC_min_out : Outport
  all_flags0.6 : Outport  Port=2
  all_flags1.6 : Outport  Port=3
  all_flags2 : Outport  Port=4
  all_range [m] : Outport  Port=5
  all_theta [deg] : Outport  Port=6
  wires:
  TIS_range [m]/1 -> TIS1 Sorting  Fun/1(TIS1range [m])
  TIS_rangedot [m/s]/1 -> TIS1 Sorting  Fun/2(TIS1rangedot [m/s])
  TIS_theta [deg]/1 -> TIS1 Sorting  Fun/3(TIS1theta [deg])
  EGO_yaw_rate_[deg/s]/1 -> Abs/1
  If/1 -> Bend road segment/Action
  Abs/1 -> If/1
  TIS1 Sorting  Fun/1(TIS1_RANGE [m]) -> Bend road segment/1(TIS_range [m]), Straight road segment/1(TIS_range [m]1), all_range [m]/1
  TIS1 Sorting  Fun/2(TIS1_RANGEDOT [m/s]) -> Bend road segment/2(TIS_rangedot [m/s]), Straight road segment/2(TIS_rangedot [m/s]1)
  TIS1 Sorting  Fun/3(TIS1_THETA [rad]) -> Bend road segment/3(TIS_theta [deg]), Straight road segment/3(TIS_theta [deg]1), Radians to Degrees/1
  If/2 -> Straight road segment/Action
  Constant2/1 -> Bend road segment/4(TTCdem1), Straight road segment/4(TTCdem1)
  Constant/1 -> Bend road segment/5(TTCdem2), Straight road segment/5(TTCdem2)
  EGO_velocity [m/s]/1 -> Bend road segment/6(EGO_velocity [m/s]1), Straight road segment/6(EGO_velocity [m/s])
  EGO_yaw_rate_[deg/s]_1/1 -> Bend road segment/7(EGO_yaw_rate_[deg/s])
  ind flag/1 -> Data Type Conversion/1
  Bend road segment/2(all_flags_0.6) -> Merge2/1
  Straight road segment/2(all_flags_0.6) -> Merge2/2
  Straight road segment/3(all_flags1.6) -> Merge3/2
  Bend road segment/3(all_flags_1.6) -> Merge3/1
  Radians to Degrees/1 -> all_theta [deg]/1
  Data Type Conversion/1 -> Logical Operator1/1
  Straight road segment/4(TTC_out) -> Merge1/2
  Bend road segment/4(TTC_out) -> Merge1/1
  Merge1/1 -> TTC_min_out/1
  Bend road segment/1(all_flags_2) -> Merge4/1
  Straight road segment/1(all_flags_2) -> Merge4/2
  Merge4/1 -> change lane/2
  Logical Operator1/1 -> change lane/1, change lane2/1, change lane1/1
  Merge3/1 -> change lane1/2
  Merge2/1 -> change lane2/2
  change lane/1 -> all_flags2/1
  change lane2/1 -> Switch/2, Switch/1
  Switch/1 -> all_flags0.6/1
  EGO_velocity [m/s]1/1 -> Compare To Constant/1
  Compare To Constant/1 -> change lane2/3, change lane1/3, change lane/3
  change lane1/1 -> all_flags1.6/1
  Data Store Read/1 -> Switch/3

== system Experiment_3_cs/Audi_A8_1/ENABLED/PPS Model/Rate transition from TIS to camera ==
  In1 : Inport
  In2 : Inport  Port=2
  In3 : Inport  Port=3
  Rate Transition1 : RateTransition  Integrity=off  Deterministic=off  X0=zeros(TISdet,1)  OutPortSampleTime=1/Camfreq
  Rate Transition2 : RateTransition  Integrity=off  Deterministic=off  X0=zeros(TISdet,1)  OutPortSampleTime=1/Camfreq
  Rate Transition3 : RateTransition  Integrity=off  Deterministic=off  X0=zeros(TISdet,1)  OutPortSampleTime=1/Camfreq
  Out1 : Outport
  Out2 : Outport  Port=2
  Out3 : Outport  Port=3
  wires:
  In1/1 -> Rate Transition3/1
  In2/1 -> Rate Transition1/1
  In3/1 -> Rate Transition2/1
  Rate Transition3/1 -> Out1/1
  Rate Transition1/1 -> Out2/1
  Rate Transition2/1 -> Out3/1

== system Experiment_3_cs/Audi_A8_1/ENABLED/PPS Model/Rate transition from main freq to TIS freq ==
  In1 : Inport
  In2 : Inport  Port=2
  Rate Transition1 : RateTransition  Integrity=off  Deterministic=off  OutPortSampleTime=1/TISfreq
  Rate Transition2 : RateTransition  Integrity=off  Deterministic=off  OutPortSampleTime=1/TISfreq
  Out1 : Outport
  Out2 : Outport  Port=2
  wires:
  Rate Transition1/1 -> Out2/1
  In2/1 -> Rate Transition1/1
  In1/1 -> Rate Transition2/1
  Rate Transition2/1 -> Out1/1

== system Experiment_3_cs/Audi_A8_1/ENABLED/PathFollower_1/CTRL REFERENCES ==
  note: REFERENCE POSITION BASED POSITION CTRL
  Pos x,y,Y [m,m,rad] : Inport
  Position Preview Distance [m] : Inport  Port=2
  TrajOffset [m,m,rad] : Inport  Port=3
  ActorOffset_Left(+) / Right(-)_[m] : Inport  Port=4
  Calculate Preview Point (pvp) by extrapolating current Vehicle Position (p0) with Preview Distance and Vehicle Orientation : Subsystem
  Demux : Demux  Outputs=[2 2]
  Demux1 : Demux  Outputs=2
  Demux2 : Demux  Outputs=2
  Find Reference Point (pref) on Trajectory closest to PVP Point (pvp) : Subsystem
      mask Display:
      | port_label('input',1,'pvp [m,m]');
      | port_label('input',2,'TrajOffset_x_y_Y [m,m,rad]');
      | port_label('input',3,'ActorOffset_Left_Right [m]');
      | port_label('input',4,'p0 [m,m,rad]');
      | port_label('output',1,'pref [m,m]');
      | port_label('output',2,'Actor_traj_distance [m]');
      | port_label('output',3,'Actor_traj_angle [m]');
  Mux1 : Mux  Inputs=2
  Reshape : Reshape  OutputDimensionality=Customize  OutputDimensions=[2,2]
  Selector1 : Selector  InputPortWidth=3  Indices=[1 2]
  Terminator : Terminator
  Terminator1 : Terminator
  Terminator2 : Terminator
  Vector Concatenate : Concatenate
  pvp  [m,m] : Outport
  pref_pvp [m,m] : Outport  Port=2
  pref_0 [m,m] : Outport  Port=3
  Actor/Traj_distance [m] : Outport  Port=4
  Actor/Traj_angle [deg] : Outport  Port=5
  wires:
  Demux1/2 -> Terminator2/1
  Demux2/2 -> Terminator1/1
  Demux1/1 -> Actor/Traj_distance [m]/1
  Demux2/1 -> Actor/Traj_angle [deg]/1
  Find Reference Point (pref) on Trajectory closest to PVP Point (pvp)/1(Out1) -> Demux/1
  Reshape/1 -> Find Reference Point (pref) on Trajectory closest to PVP Point (pvp)/1(In1)
  Vector Concatenate/1 -> Reshape/1
  Mux1/1 -> Vector Concatenate/2, pvp  [m,m]/1
  Pos x,y,Y [m,m,rad]/1 -> Calculate Preview Point (pvp) by extrapolating current Vehicle Position (p0) with Preview Distance and Vehicle Orientation/2(x,y,Y Demux [m,m,rad]), Find Reference Point (pref) on Trajectory closest to PVP Point (pvp)/4(In4), Selector1/1
  Calculate Preview Point (pvp) by extrapolating current Vehicle Position (p0) with Preview Distance and Vehicle Orientation/1(x_glob_PVD) -> Mux1/1
  Calculate Preview Point (pvp) by extrapolating current Vehicle Position (p0) with Preview Distance and Vehicle Orientation/3(Y [rad]) -> Terminator/1
  Position Preview Distance [m]/1 -> Calculate Preview Point (pvp) by extrapolating current Vehicle Position (p0) with Preview Distance and Vehicle Orientation/1(Preview Distance)
  Demux/2 -> pref_pvp [m,m]/1
  Demux/1 -> pref_0 [m,m]/1
  Calculate Preview Point (pvp) by extrapolating current Vehicle Position (p0) with Preview Distance and Vehicle Orientation/2(y_glob_PVD) -> Mux1/2
  TrajOffset [m,m,rad]/1 -> Find Reference Point (pref) on Trajectory closest to PVP Point (pvp)/2(In2)  "L6"
  ActorOffset_Left(+) / Right(-)_[m]/1 -> Find Reference Point (pref) on Trajectory closest to PVP Point (pvp)/3(In3)
  Selector1/1 -> Vector Concatenate/1
  Find Reference Point (pref) on Trajectory closest to PVP Point (pvp)/2(Out2) -> Demux1/1
  Find Reference Point (pref) on Trajectory closest to PVP Point (pvp)/3(Out3) -> Demux2/1

== system Experiment_3_cs/Audi_A8_1/ENABLED/PathFollower_1/Calculate shifted p0 wrt COG ==
  position x,y,Y [m,m,deg] : Inport
  Constant1 : Constant  Value=XShifting_wrt_COG
  Degrees to Radians : simulink_extras/Transformations/Degrees to Radians
  Demux1 : Demux  Outputs=3
  Fcn : Fcn  Expr=u(2)*cos(u(1))
  Fcn1 : Fcn  Expr=u(2)*sin(u(1))
  Mux1 : Mux  Inputs=3
  Mux2 : Mux  Inputs=2
  Sum : Sum  Inputs=|++
  Sum1 : Sum  Inputs=|++
  position x,y,Y [m,m,rad] : Outport
  wires:
  Sum/1 -> Mux1/1
  Sum1/1 -> Mux1/2
  Demux1/1 -> Sum/1
  Demux1/3 -> Degrees to Radians/1
  Degrees to Radians/1 -> Mux2/1, Mux1/3
  Mux2/1 -> Fcn/1, Fcn1/1
  Fcn/1 -> Sum/2
  Fcn1/1 -> Sum1/2
  Demux1/2 -> Sum1/1
  position x,y,Y [m,m,deg]/1 -> Demux1/1
  Mux1/1 -> position x,y,Y [m,m,rad]/1
  Constant1/1 -> Mux2/2
